simulink model "untitled"  (R2023b)
settings: Solver=VariableStepAuto  StartTime=0.0  StopTime=10  RelTol=1e-3
settings Model: Creator=CL605_08  LastModifiedBy=CL605_08

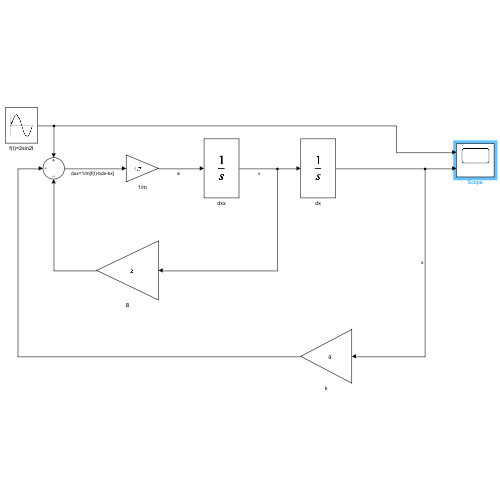
[thumbnail: Simulink's stored preview of the top-level diagram]
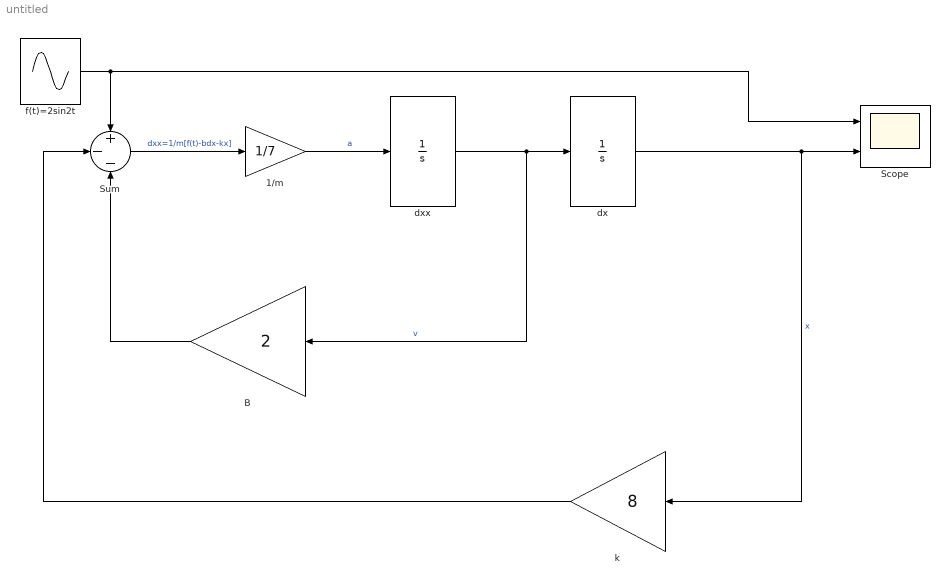
== system untitled ==
  1/m : Gain  Gain=1/7
  B : Gain  Gain=2
  Scope : Scope  NumInputPorts=2
  Sum : Sum  Inputs=+--
  dx : Integrator
  dxx : Integrator
  f(t)=2sin2t : Sin  Amplitude=2  Frequency=2  SampleTime=0
  k : Gain  Gain=8
  wires:
  dxx/1 -> B/1, dx/1  "v"
  1/m/1 -> dxx/1  "a"
  Sum/1 -> 1/m/1  "dxx=1/m[f(t)-bdx-kx]"
  dx/1 -> k/1, Scope/2  "x"
  B/1 -> Sum/3
  k/1 -> Sum/2
  f(t)=2sin2t/1 -> Scope/1, Sum/1
